simulink model "FourBitAdder"  (R2024a)
settings: Solver=ode45  StartTime=0.0  StopTime=inf  RelTol=1e-3  EnableMultiTasking=on
settings Model: Creator=nunkesser  LastModifiedBy=nunkesser
settings SolverCC: AlgebraicLoopSolver=TrustRegion
settings DataIOCC: LimitDataPoints=on  SaveFormat=Array  ReturnWorkspaceOutputs=off
settings OptimizationCC: LifeSpan=inf
settings DebuggingCC: SolverPrmCheckMsg=warning  UnconnectedInputMsg=warning  UnconnectedOutputMsg=warning  UnconnectedLineMsg=warning  SFUnexpectedBacktrackingDiag=warning  SFNoUnconditionalDefaultTransitionDiag=warning  SFExecutionAtInitializationDiag=none  ArithmeticOperatorsInVariantConditions=warning
settings HardwareCC: ProdBitPerPointer=32  ProdBitPerSizeT=32  ProdBitPerPtrDiffT=32  ProdLargestAtomicFloat=None  ProdIntDivRoundTo=Undefined  ProdEndianess=Unspecified  ProdWordSize=32  ProdHWDeviceType=32-bit Generic
settings ModelReferenceCC: PropagateSignalLabelsOutOfModel=off
settings SFSimCC: SimUseLocalCustomCode=off  CustomCodeUndefinedFunction=UseInterfaceOnly
settings RTWCC: RTWUseLocalCustomCode=off  GPUComputeCapability=3.5
settings CodeAppCC: StateflowObjectComments=on
settings GRTTargetCC: TargetLangStandard=C89/C90 (ANSI)
settings ConfigComp: CovMetricSettings=dw  CovSaveCumulativeToWorkspaceVar=on  CovSaveSingleToWorkspaceVar=on  CovExternalEMLEnable=off  CovSFcnEnable=off

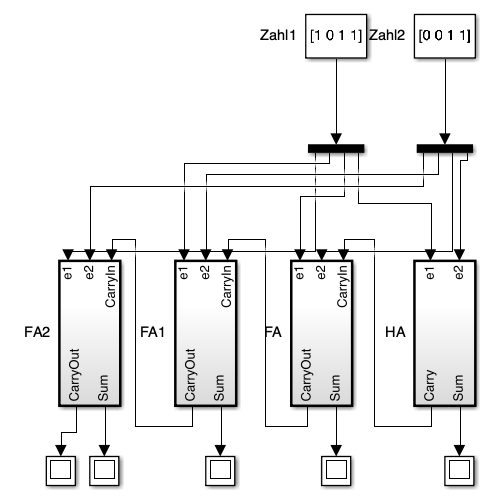
[thumbnail: Simulink's stored preview of the top-level diagram]
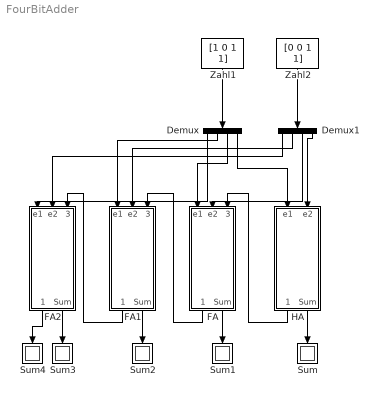
== system FourBitAdder ==
  Demux : Demux
  Demux1 : Demux
  FA : Subsystem  TreatAsAtomicUnit=on
  FA1 : Subsystem  TreatAsAtomicUnit=on
  FA2 : Subsystem  TreatAsAtomicUnit=on
  HA : Subsystem  TreatAsAtomicUnit=on
  Sum{,1..4} (5 alike) : Display
  Zahl1 : Constant  Value=[1 0 1 1]
  Zahl2 : Constant  Value=[0 0 1 1]
  wires:
  Zahl1/1 -> Demux/1
  Demux/4 -> HA/1(e1)
  Zahl2/1 -> Demux1/1
  HA/2(Sum) -> Sum/1
  HA/1(Carry) -> FA/3(CarryIn)
  Demux1/4 -> HA/2(e2)
  FA/2(Sum) -> Sum1/1
  Demux1/3 -> FA/2(e2)
  Demux/3 -> FA/1(e1)
  FA/1(CarryOut) -> FA1/3(CarryIn)
  Demux1/2 -> FA1/2(e2)
  Demux/2 -> FA1/1(e1)
  FA1/2(Sum) -> Sum2/1
  FA1/1(CarryOut) -> FA2/3(CarryIn)
  Demux/1 -> FA2/1(e1)
  Demux1/1 -> FA2/2(e2)
  FA2/2(Sum) -> Sum3/1
  FA2/1(CarryOut) -> Sum4/1

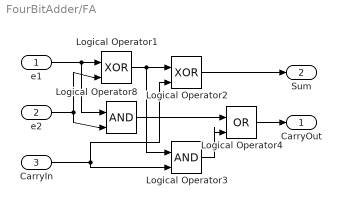
== system FourBitAdder/FA ==
  e1 : Inport
  e2 : Inport  Port=2
  CarryIn : Inport  Port=3
  Logical Operator1 : Logic  Operator=XOR  IconShape=distinctive  AllPortsSameDT=off  OutDataTypeStr=boolean
  Logical Operator2 : Logic  Operator=XOR  IconShape=distinctive  AllPortsSameDT=off  OutDataTypeStr=boolean
  Logical Operator3 : Logic  IconShape=distinctive  AllPortsSameDT=off  OutDataTypeStr=boolean
  Logical Operator4 : Logic  Operator=OR  IconShape=distinctive  AllPortsSameDT=off  OutDataTypeStr=boolean
  Logical Operator8 : Logic  IconShape=distinctive  AllPortsSameDT=off  OutDataTypeStr=boolean
  CarryOut : Outport
  Sum : Outport  Port=2
  wires:
  e2/1 -> Logical Operator8/2, Logical Operator1/2
  Logical Operator1/1 -> Logical Operator2/1, Logical Operator3/1
  CarryIn/1 -> Logical Operator2/2, Logical Operator3/2
  Logical Operator2/1 -> Sum/1
  Logical Operator8/1 -> Logical Operator4/1
  Logical Operator3/1 -> Logical Operator4/2
  Logical Operator4/1 -> CarryOut/1
  e1/1 -> Logical Operator8/1, Logical Operator1/1

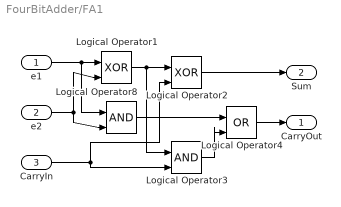
== system FourBitAdder/FA1 ==
  e1 : Inport
  e2 : Inport  Port=2
  CarryIn : Inport  Port=3
  Logical Operator1 : Logic  Operator=XOR  IconShape=distinctive  AllPortsSameDT=off  OutDataTypeStr=boolean
  Logical Operator2 : Logic  Operator=XOR  IconShape=distinctive  AllPortsSameDT=off  OutDataTypeStr=boolean
  Logical Operator3 : Logic  IconShape=distinctive  AllPortsSameDT=off  OutDataTypeStr=boolean
  Logical Operator4 : Logic  Operator=OR  IconShape=distinctive  AllPortsSameDT=off  OutDataTypeStr=boolean
  Logical Operator8 : Logic  IconShape=distinctive  AllPortsSameDT=off  OutDataTypeStr=boolean
  CarryOut : Outport
  Sum : Outport  Port=2
  wires:
  e2/1 -> Logical Operator8/2, Logical Operator1/2
  Logical Operator1/1 -> Logical Operator2/1, Logical Operator3/1
  CarryIn/1 -> Logical Operator2/2, Logical Operator3/2
  Logical Operator2/1 -> Sum/1
  Logical Operator8/1 -> Logical Operator4/1
  Logical Operator3/1 -> Logical Operator4/2
  Logical Operator4/1 -> CarryOut/1
  e1/1 -> Logical Operator8/1, Logical Operator1/1

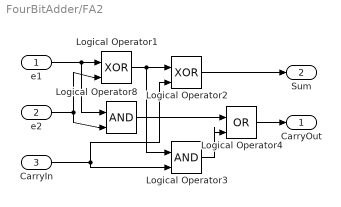
== system FourBitAdder/FA2 ==
  e1 : Inport
  e2 : Inport  Port=2
  CarryIn : Inport  Port=3
  Logical Operator1 : Logic  Operator=XOR  IconShape=distinctive  AllPortsSameDT=off  OutDataTypeStr=boolean
  Logical Operator2 : Logic  Operator=XOR  IconShape=distinctive  AllPortsSameDT=off  OutDataTypeStr=boolean
  Logical Operator3 : Logic  IconShape=distinctive  AllPortsSameDT=off  OutDataTypeStr=boolean
  Logical Operator4 : Logic  Operator=OR  IconShape=distinctive  AllPortsSameDT=off  OutDataTypeStr=boolean
  Logical Operator8 : Logic  IconShape=distinctive  AllPortsSameDT=off  OutDataTypeStr=boolean
  CarryOut : Outport
  Sum : Outport  Port=2
  wires:
  e2/1 -> Logical Operator8/2, Logical Operator1/2
  Logical Operator1/1 -> Logical Operator2/1, Logical Operator3/1
  CarryIn/1 -> Logical Operator2/2, Logical Operator3/2
  Logical Operator2/1 -> Sum/1
  Logical Operator8/1 -> Logical Operator4/1
  Logical Operator3/1 -> Logical Operator4/2
  Logical Operator4/1 -> CarryOut/1
  e1/1 -> Logical Operator8/1, Logical Operator1/1

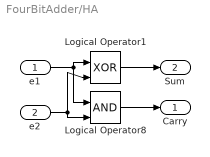
== system FourBitAdder/HA ==
  e1 : Inport
  e2 : Inport  Port=2
  Logical Operator1 : Logic  Operator=XOR  IconShape=distinctive  AllPortsSameDT=off  OutDataTypeStr=boolean
  Logical Operator8 : Logic  IconShape=distinctive  AllPortsSameDT=off  OutDataTypeStr=boolean
  Carry : Outport
  Sum : Outport  Port=2
  wires:
  e1/1 -> Logical Operator1/1, Logical Operator8/1
  e2/1 -> Logical Operator1/2, Logical Operator8/2
  Logical Operator1/1 -> Sum/1
  Logical Operator8/1 -> Carry/1
